simulink model "sampleModel20"  (R2021a)
settings: Solver=VariableStepAuto  StartTime=0.0  StopTime=10.0  RelTol=1e-3
undefined symbols (not defined in the file): DiscIntNeverNeededParam, magnitude, Newton, Raphson
libraries: simulink x274, pid_lib x17
(part 1 of 16)
settings Model: Creator=user  LastModifiedBy=user

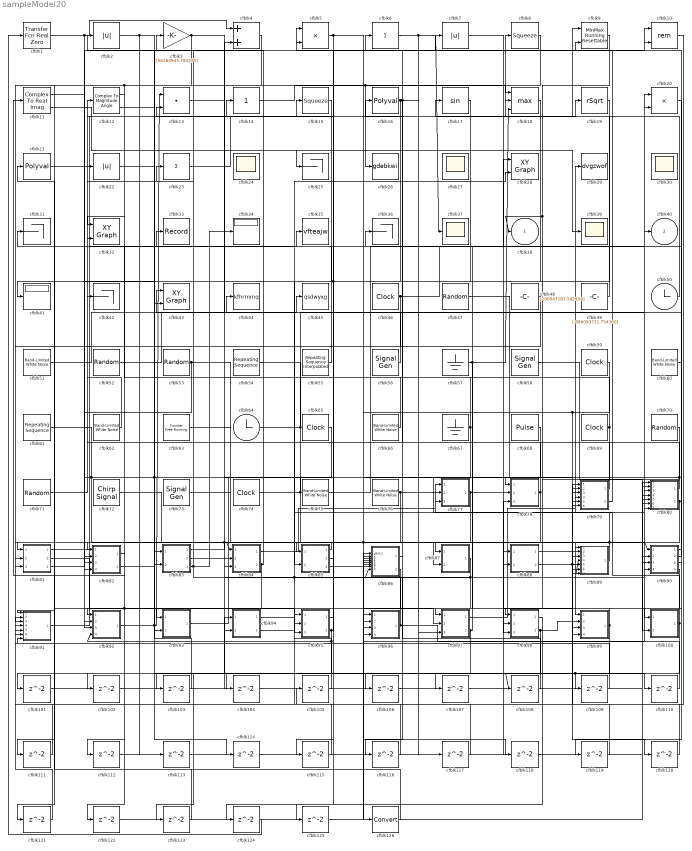
== system sampleModel20 ==
  cfblk1 : simulink/Discrete/Transfer Fcn Real Zero  ZeroZ=0.75  ICPrevInput=0.0  DoSatur=off
      settings: SourceProductBaseCode=SL
  cfblk10 : Math  Operator=rem  SaturateOnIntegerOverflow=on
  cfblk100 : Subsystem
  cfblk{101..125} (25 alike) : Delay  SampleTime=1
  cfblk11 : ComplexToRealImag
  cfblk12 : ComplexToMagnitudeAngle
  cfblk126 : DataTypeConversion
  cfblk13 : DotProduct  InputSameDT=on  OutDataTypeStr=Inherit: Inherit via internal rule
  cfblk14 : simulink/Math Operations/Slider Gain  gain=1  low=0  high=2
  cfblk15 : Squeeze
  cfblk16 : Polyval  Coefs=[ +2.081618890e-019, -1.441693666e-014, +4.719686976e-010, -8.536869453e-006, +1.621573104e-001, -8.087801117e+001 ]
  cfblk17 : Trigonometry
  cfblk18 : MinMax  Function=max  Inputs=3
  cfblk19 : Sqrt  Operator=rSqrt  AlgorithmType=Newton-Raphson  SaturateOnIntegerOverflow=on
  cfblk2 : Abs
  cfblk20 : Product  Inputs=**
  cfblk21 : Polyval  Coefs=[ +2.081618890e-019, -1.441693666e-014, +4.719686976e-010, -8.536869453e-006, +1.621573104e-001, -8.087801117e+001 ]
  cfblk22 : Abs
  cfblk23 : Sum  Inputs=+
  cfblk{24,27,30,37,39} (5 alike) : Scope
      cfblk24 settings: Floating=on
      cfblk27 settings: Floating=on
      cfblk30 settings: Floating=on
  cfblk{25,31,36,42} (4 alike) : Terminator
  cfblk26 : ToWorkspace  VariableName=gdebkwi  SaveFormat=Timeseries  SampleTime=-1
  cfblk28 : simulink/Sinks/XY Graph  xmin=-1  xmax=1  ymin=-1  ymax=1  st=-1
  cfblk29 : ToWorkspace  VariableName=dvgzwof  SaveFormat=Timeseries  SampleTime=-1
  cfblk3 : Gain  Gain=[56264945.784275]
  cfblk32 : simulink/Sinks/XY Graph  xmin=-1  xmax=1  ymin=-1  ymax=1  st=-1
  cfblk33 : Record  FileSettingsInternal="{\"entries\":[{\"content\":{\"excelSettings\":{\"content\":{},\"type\":\"Streamout.ExcelSettings\"}},\"type\":\"Streamout.FileSettingStorage\",\"uuid\":\"928b06ce-2ca3-4e43-b9c9-2fca8fc53509\"}],\"packageUris\":[\"http://schema.mathworks.com/mf0/streamout_blocks/R2020a\"],\"version\":\"1.0\"}"  SignalsInternal="{\"entries\":[{\"content\":{\"signals\":[{\"content\":{\"blockPath\":[\"sampleModel20/cfblk33\"],\"channel\":[],\"dimensions\":[1],\"domain\":\"samplemodel20/cfblk33\",\"lineColor\":\"#77ac30\",\"plots\":[1],\"port\":1,\"sid\":[\"\"],\"signalID\":19970752,\"signalName\":\"cfblk55\"},\"type\":\"RecordBlkView.Signal\",\"uuid\":\"c558b8a0-6107-4ffd-af5c-dee7680296d7\"}]},\"type\":\"RecordBlkView.InputSignals\",\"uuid\":\"2b2755c9-adf7-49b9-84f7-e9e1f548de1f\"}],\"packageUris\":[\"http://schema.mathworks.com/mf0/streamout_blocks/R2020a\"],\"version\":\"1.0\"}"  VisualizationBindings="{\"sparklinesplugin\":{\"info\":[{\"bindingParametersList\":[],\"subplotID\":1}]}}"
  cfblk34 : Display
  cfblk35 : ToWorkspace  VariableName=vfteajw  SaveFormat=Timeseries  SampleTime=-1
  cfblk4 : Sum
  cfblk41 : Display
  cfblk43 : simulink/Sinks/XY Graph  xmin=-1  xmax=1  ymin=-1  ymax=1  st=-1
  cfblk44 : ToWorkspace  VariableName=kfhrmmq  SaveFormat=Timeseries  SampleTime=-1
  cfblk45 : ToWorkspace  VariableName=qsdwyxg  SaveFormat=Timeseries  SampleTime=-1
  cfblk{46,59,65,69,74} (5 alike) : DigitalClock
  cfblk47 : RandomNumber  Mean=[-41753.040388]  Variance=[63915.709445]  Seed=[511170235.000000]  SampleTime=0.1
  cfblk48 : Constant  Value=[200047183.582154]  SampleTime=1
  cfblk49 : Constant  Value=[-886093721.754360]  SampleTime=1
  cfblk5 : Product
  cfblk50 : Clock
  cfblk51 : simulink/Sources/Band-Limited White Noise  Cov=[9193384842.285128]  Ts=0.1  seed=[7756507675.000000]
  cfblk52 : RandomNumber  Mean=[-72813.346888]  Variance=[96356.026322]  Seed=[58960493.000000]  SampleTime=0.1
  cfblk53 : UniformRandomNumber  Minimum=[-6749666358.615873]  Maximum=[6273327936.656572]  Seed=[6207066.000000]  SampleTime=0.1
  cfblk54 : simulink/Sources/Repeating Sequence  rep_seq_t=[0 2]  rep_seq_y=[334719478.211440, -569550998.056046]
  cfblk55 : simulink/Sources/Repeating Sequence Interpolated  OutValues=[101544910.946823, 391282082.256712, 433310399.263298, 204880323.228426, -388511505.652922]  TimeValues=[0 0.1 0.5 0.6 1].'  LookUpMeth=Use Input Nearest  tsamp=0.01  OutMin=[]  OutMax=[]  OutDataTypeStr=double  OutputDataTypeScalingMode=double  OutDataType=fixdt(0,8)  OutScaling=2^-10
  cfblk56 : SignalGenerator  WaveForm=square  Amplitude=[548376924.788326]
  cfblk57 : Ground
  cfblk58 : SignalGenerator  Amplitude=[184204147.684020]
  cfblk6 : Sum  Inputs=+
  cfblk60 : simulink/Sources/Band-Limited White Noise  Cov=[6011912995.701045]  Ts=0.1  seed=[7883111785.000000]
  cfblk61 : simulink/Sources/Repeating Sequence  rep_seq_t=[0 2]  rep_seq_y=[573110201.455736, -888529698.256362]
  cfblk62 : simulink/Sources/Band-Limited White Noise  Cov=[5852828294.400876]  Ts=0.1  seed=[308601692.000000]
  cfblk63 : simulink/Sources/Counter Free-Running  NumBits=[57.000000]  tsamp=-1
  cfblk64 : Clock
  cfblk66 : simulink/Sources/Band-Limited White Noise  Cov=[6955568622.597345]  Ts=0.1  seed=[820560845.000000]
  cfblk67 : Ground
  cfblk68 : DiscretePulseGenerator  PulseType=Time based  Amplitude=[-307176578.790476]  Period=[8696334.995462]  PulseWidth=5  PhaseDelay=[9.000000]
  cfblk7 : Abs
  cfblk70 : UniformRandomNumber  Minimum=[-759248775.546139]  Maximum=[9415666302.746086]  Seed=[58100389.000000]  SampleTime=0.1
  cfblk71 : UniformRandomNumber  Minimum=[-2486475271.173175]  Maximum=[2075060491.074587]  Seed=[20322190.000000]  SampleTime=0.1
  cfblk72 : simulink/Sources/Chirp Signal  f1=[314613710.646437]  T=[-916076924.706605]  f2=[-822624780.040317]
  cfblk73 : SignalGenerator  Amplitude=[415883044.932598]  Units=rad/sec
  cfblk75 : simulink/Sources/Band-Limited White Noise  Cov=[1094535168.541819]  Ts=0.1  seed=[4220656770.000000]
  cfblk76 : simulink/Sources/Band-Limited White Noise  Cov=[7039707520.686424]  Ts=0.1  seed=[3381655650.000000]
  cfblk77 : Subsystem
  cfblk78 : Subsystem
  cfblk79 : Subsystem
  cfblk8 : Squeeze
  cfblk80 : Subsystem
  cfblk81 : Subsystem
  cfblk82 : Subsystem
  cfblk83 : Subsystem
  cfblk84 : Subsystem
  cfblk85 : Subsystem
  cfblk86 : Subsystem
  cfblk87 : Subsystem
  cfblk88 : Subsystem
  cfblk89 : Subsystem
  cfblk9 : simulink/Math Operations/MinMax Running Resettable  Function=min  vinit=0.0
  cfblk90 : Subsystem
  cfblk91 : Subsystem
  cfblk92 : Subsystem
  cfblk93 : Subsystem
  cfblk94 : Subsystem
  cfblk95 : Subsystem
  cfblk96 : Subsystem
  cfblk97 : Subsystem
  cfblk98 : Subsystem
  cfblk99 : Subsystem
  cfblk38 : Outport
  cfblk40 : Outport  Port=2
  wires:
  cfblk74/1 -> cfblk99/1(cfblk1), cfblk79/2(cfblk10)
  cfblk93/1(cfblk2) -> cfblk78/1(cfblk1)
  cfblk96/1(cfblk2) -> cfblk20/1, cfblk3/1
  cfblk90/1(cfblk2) -> cfblk5/1
  cfblk50/1 -> cfblk8/1
  cfblk81/1(cfblk2) -> cfblk35/1
  cfblk8/1 -> cfblk26/1, cfblk81/3(cfblk9)
  cfblk6/1 -> cfblk37/1, cfblk97/3(cfblk6)
  cfblk84/1(cfblk2) -> cfblk77/1(cfblk1)
  cfblk49/1 -> cfblk17/1
  cfblk1/1 -> cfblk4/1, cfblk79/5(cfblk13)
  cfblk71/1 -> cfblk15/1
  cfblk62/1 -> cfblk12/1
  cfblk64/1 -> cfblk20/2, cfblk98/2(cfblk10)
  cfblk3/1 -> cfblk111/1, cfblk112/1, cfblk89/7(cfblk15), cfblk110/1
  cfblk15/1 -> cfblk41/1
  cfblk90/2(cfblk13) -> cfblk36/1
  cfblk84/2(cfblk13) -> cfblk121/1, cfblk122/1, cfblk2/1
  cfblk82/1(cfblk2) -> cfblk11/1
  cfblk92/1(cfblk2) -> cfblk13/1, cfblk107/1
  cfblk87/1(cfblk2) -> cfblk86/8(cfblk16), cfblk102/1
  cfblk67/1 -> cfblk5/2, cfblk86/5(cfblk13)
  cfblk73/1 -> cfblk90/1(cfblk1), cfblk86/4(cfblk12)
  cfblk91/1(cfblk2) -> cfblk19/1
  cfblk56/1 -> cfblk44/1
  cfblk55/1 -> cfblk33/1
  cfblk79/1(cfblk2) -> cfblk16/1
  cfblk89/1(cfblk2) -> cfblk84/1(cfblk1), cfblk79/4(cfblk12)
  cfblk20/1 -> cfblk100/1(cfblk1)
  cfblk4/1 -> cfblk94/2(cfblk12)
  cfblk66/1 -> cfblk23/1
  cfblk85/1(cfblk2) -> cfblk82/1(cfblk1)
  cfblk18/1 -> cfblk96/2(cfblk8)
  cfblk58/1 -> cfblk100/2(cfblk12)
  cfblk52/1 -> cfblk45/1
  cfblk5/1 -> cfblk85/1(cfblk1), cfblk97/2(cfblk5)
  cfblk85/2(cfblk12) -> cfblk13/2
  cfblk23/1 -> cfblk9/1
  cfblk68/1 -> cfblk87/1(cfblk1)
  cfblk99/1(cfblk2) -> cfblk108/1, cfblk109/1, cfblk92/1(cfblk1)
  cfblk97/1(cfblk2) -> cfblk29/1
  cfblk53/1 -> cfblk92/2(cfblk5), cfblk98/3(cfblk11)
  cfblk14/1 -> cfblk18/1
  cfblk46/1 -> cfblk40/1, cfblk91/3(cfblk10)
  cfblk72/1 -> cfblk89/1(cfblk1)
  cfblk78/1(cfblk2) -> cfblk42/1, cfblk81/2(cfblk8)
  cfblk16/1 -> cfblk82/4(cfblk7), cfblk115/1, cfblk116/1, cfblk117/1
  cfblk97/2(cfblk7) -> cfblk31/1, cfblk101/1
  cfblk60/1 -> cfblk10/1
  cfblk21/1 -> cfblk18/2
  cfblk80/1(cfblk2) -> cfblk6/1
  cfblk57/1 -> cfblk18/3, cfblk97/1(cfblk1)
  cfblk70/1 -> cfblk93/1(cfblk1), cfblk88/2(cfblk7)
  cfblk17/1 -> cfblk85/2(cfblk11)
  cfblk59/1 -> cfblk89/5(cfblk13), cfblk89/6(cfblk14), cfblk96/4(cfblk10)
  cfblk12/1 -> cfblk32/1
  cfblk54/1 -> cfblk78/2(cfblk11)
  cfblk9/1 -> cfblk38/1, cfblk98/1(cfblk1)
  cfblk69/1 -> cfblk32/2, cfblk79/3(cfblk11)
  cfblk65/1 -> cfblk84/2(cfblk11)
  cfblk86/1(cfblk2) -> cfblk93/2(cfblk8)
  cfblk81/2(cfblk10) -> cfblk95/3(cfblk13)
  cfblk79/2(cfblk15) -> cfblk7/1
  cfblk51/1 -> cfblk4/2
  cfblk88/1(cfblk2) -> cfblk90/3(cfblk11)
  cfblk22/1 -> cfblk84/3(cfblk12)
  cfblk81/3(cfblk11) -> cfblk9/2
  cfblk75/1 -> cfblk28/1
  cfblk12/2 -> cfblk25/1
  cfblk2/1 -> cfblk79/6(cfblk14), cfblk114/1, cfblk113/1
  cfblk98/2(cfblk12) -> cfblk99/2(cfblk8), cfblk125/1
  cfblk80/2(cfblk13) -> cfblk43/1, cfblk91/1(cfblk1)
  cfblk19/1 -> cfblk83/2(cfblk8)
  cfblk83/1(cfblk2) -> cfblk87/2(cfblk10)
  cfblk76/1 -> cfblk81/1(cfblk1), cfblk80/7(cfblk12)
  cfblk61/1 -> cfblk89/2(cfblk10), cfblk77/2(cfblk11)
  cfblk90/4(cfblk15) -> cfblk99/3(cfblk9)
  cfblk95/2(cfblk14) -> cfblk92/4(cfblk7), cfblk123/1, cfblk14/1
  cfblk82/2(cfblk8) -> cfblk10/2
  cfblk100/1(cfblk2) -> cfblk77/3(cfblk12), cfblk104/1
  cfblk77/1(cfblk2) -> cfblk82/2(cfblk5), cfblk99/4(cfblk10)
  cfblk48/1 -> cfblk82/3(cfblk6)
  cfblk47/1 -> cfblk89/3(cfblk11)
  cfblk7/1 -> cfblk88/1(cfblk1)
  cfblk83/2(cfblk9) -> cfblk90/4(cfblk12)
  cfblk94/1(cfblk2) -> cfblk80/3(cfblk8)
  cfblk94/2(cfblk13) -> cfblk28/2, cfblk89/4(cfblk12)
  cfblk86/2(cfblk17) -> cfblk92/3(cfblk6)
  cfblk83/3(cfblk10) -> cfblk22/1, cfblk34/1
  cfblk11/1 -> cfblk43/2
  cfblk11/2 -> cfblk39/1
  cfblk101/1 -> cfblk80/4(cfblk9)
  cfblk102/1 -> cfblk94/1(cfblk1)
  cfblk95/1(cfblk2) -> cfblk103/1
  cfblk103/1 -> cfblk83/1(cfblk1)
  cfblk104/1 -> cfblk86/1(cfblk1)
  cfblk10/1 -> cfblk105/1
  cfblk105/1 -> cfblk95/1(cfblk1)
  cfblk13/1 -> cfblk106/1
  cfblk106/1 -> cfblk80/1(cfblk1)
  cfblk107/1 -> cfblk80/5(cfblk10)
  cfblk108/1 -> cfblk86/3(cfblk11)
  cfblk109/1 -> cfblk91/6(cfblk13)
  cfblk110/1 -> cfblk96/1(cfblk1)
  cfblk111/1 -> cfblk91/2(cfblk9)
  cfblk112/1 -> cfblk86/6(cfblk14)
  cfblk113/1 -> cfblk80/2(cfblk7)
  cfblk114/1 -> cfblk78/3(cfblk12)
  cfblk115/1 -> cfblk95/2(cfblk12)
  cfblk116/1 -> cfblk86/2(cfblk10)
  cfblk117/1 -> cfblk91/5(cfblk12)
  cfblk85/3(cfblk13) -> cfblk118/1
  cfblk118/1 -> cfblk90/2(cfblk10)
  cfblk90/3(cfblk14) -> cfblk119/1
  cfblk119/1 -> cfblk96/3(cfblk9)
  cfblk88/2(cfblk8) -> cfblk120/1
  cfblk120/1 -> cfblk79/1(cfblk1)
  cfblk121/1 -> cfblk91/4(cfblk11)
  cfblk122/1 -> cfblk80/6(cfblk11)
  cfblk123/1 -> cfblk91/7(cfblk14)
  cfblk98/1(cfblk2) -> cfblk124/1
  cfblk124/1 -> cfblk1/1
  cfblk125/1 -> cfblk86/7(cfblk15)
  cfblk63/1 -> cfblk126/1
  cfblk126/1 -> cfblk21/1

== system sampleModel20/cfblk100 ==
  cfblk1 : Inport
  cfblk12 : Inport  Port=2
  cfblk10 : Subsystem
  cfblk11 : Subsystem
  cfblk{13..19} (7 alike) : Delay  SampleTime=1
  cfblk3 : DiscreteFir  SampleTime=1
  cfblk4 : Product
  cfblk5 : Bias  Bias=[44627423.710003]
  cfblk6 : Sin  TimeSource=Use external signal  SampleTime=0
  cfblk7 : Subsystem
  cfblk8 : Subsystem
  cfblk9 : Subsystem
  cfblk2 : Outport
  wires:
  cfblk7/1(cfblk2) -> cfblk5/1
  cfblk1/1 -> cfblk7/1(cfblk1), cfblk8/2(cfblk11)
  cfblk12/1 -> cfblk10/1(cfblk1)
  cfblk5/1 -> cfblk6/1, cfblk11/2(cfblk9)
  cfblk9/1(cfblk2) -> cfblk3/1
  cfblk3/1 -> cfblk8/3(cfblk12), cfblk18/1
  cfblk9/2(cfblk12) -> cfblk4/1, cfblk19/1
  cfblk8/1(cfblk2) -> cfblk2/1, cfblk17/1
  cfblk6/1 -> cfblk11/1(cfblk1), cfblk10/2(cfblk4), cfblk15/1, cfblk16/1
  cfblk4/1 -> cfblk8/1(cfblk1)
  cfblk11/1(cfblk2) -> cfblk13/1, cfblk14/1
  cfblk10/1(cfblk2) -> cfblk4/2
  cfblk10/2(cfblk6) -> cfblk9/2(cfblk10)
  cfblk10/3(cfblk7) -> cfblk9/3(cfblk11)
  cfblk13/1 -> cfblk7/3(cfblk5)
  cfblk14/1 -> cfblk7/6(cfblk8)
  cfblk15/1 -> cfblk7/4(cfblk6)
  cfblk16/1 -> cfblk7/5(cfblk7)
  cfblk17/1 -> cfblk7/2(cfblk4)
  cfblk18/1 -> cfblk9/1(cfblk1)
  cfblk19/1 -> cfblk10/3(cfblk5)

== system sampleModel20/cfblk77 ==
  cfblk1 : Inport
  cfblk11 : Inport  Port=2
  cfblk12 : Inport  Port=3
  cfblk10 : Subsystem
  cfblk{13..23} (11 alike) : Delay  SampleTime=1
  cfblk3 : Polyval  Coefs=[ +2.081618890e-019, -1.441693666e-014, +4.719686976e-010, -8.536869453e-006, +1.621573104e-001, -8.087801117e+001 ]
  cfblk4 : Subsystem
  cfblk5 : Subsystem
  cfblk6 : Subsystem
  cfblk7 : Subsystem
  cfblk8 : Subsystem
  cfblk9 : Subsystem
  cfblk2 : Outport
  wires:
  cfblk9/1(cfblk2) -> cfblk5/4(cfblk13), cfblk13/1
  cfblk10/1(cfblk2) -> cfblk4/3(cfblk8), cfblk20/1, cfblk21/1
  cfblk4/1(cfblk2) -> cfblk17/1, cfblk18/1, cfblk19/1
  cfblk8/1(cfblk2) -> cfblk7/1(cfblk1)
  cfblk11/1 -> cfblk7/2(cfblk11), cfblk5/5(cfblk14)
  cfblk6/1(cfblk2) -> cfblk2/1, cfblk9/4(cfblk10), cfblk5/3(cfblk12)
  cfblk7/1(cfblk2) -> cfblk4/2(cfblk7), cfblk16/1
  cfblk3/1 -> cfblk10/1(cfblk1)
  cfblk12/1 -> cfblk8/2(cfblk11), cfblk8/4(cfblk13), cfblk5/1(cfblk1)
  cfblk5/3(cfblk17) -> cfblk8/3(cfblk12), cfblk23/1
  cfblk8/2(cfblk14) -> cfblk4/1(cfblk1)
  cfblk1/1 -> cfblk6/3(cfblk11)
  cfblk8/3(cfblk15) -> cfblk10/2(cfblk8), cfblk3/1, cfblk22/1
  cfblk13/1 -> cfblk6/1(cfblk1)
  cfblk5/1(cfblk2) -> cfblk14/1
  cfblk14/1 -> cfblk9/1(cfblk1)
  cfblk5/2(cfblk16) -> cfblk15/1
  cfblk15/1 -> cfblk9/3(cfblk9)
  cfblk16/1 -> cfblk8/1(cfblk1)
  cfblk17/1 -> cfblk6/2(cfblk10)
  cfblk18/1 -> cfblk6/4(cfblk12)
  cfblk19/1 -> cfblk5/2(cfblk11)
  cfblk20/1 -> cfblk9/2(cfblk8)
  cfblk21/1 -> cfblk9/5(cfblk11)
  cfblk22/1 -> cfblk5/6(cfblk15)
  cfblk23/1 -> cfblk6/5(cfblk13)

== system sampleModel20/cfblk78 ==
  cfblk1 : Inport
  cfblk11 : Inport  Port=2
  cfblk12 : Inport  Port=3
  cfblk10 : Subsystem
  cfblk{13..17} (5 alike) : Delay  SampleTime=1
  cfblk3 : simulink/Math Operations/MinMax Running Resettable  Function=min  vinit=0.0
  cfblk4 : Gain  Gain=[460184009.400901]
  cfblk5 : Sum  Inputs=+-
  cfblk6 : Product  Inputs=*
  cfblk7 : Subsystem
  cfblk8 : Subsystem
  cfblk9 : Subsystem
  cfblk2 : Outport
  wires:
  cfblk5/1 -> cfblk10/1(cfblk1)
  cfblk12/1 -> cfblk6/1, cfblk8/3(cfblk8), cfblk5/2
  cfblk9/1(cfblk2) -> cfblk7/1(cfblk1)
  cfblk11/1 -> cfblk2/1, cfblk5/1
  cfblk10/1(cfblk2) -> cfblk3/1
  cfblk1/1 -> cfblk7/2(cfblk8), cfblk10/3(cfblk10)
  cfblk8/1(cfblk2) -> cfblk3/2, cfblk14/1
  cfblk6/1 -> cfblk10/2(cfblk9), cfblk10/5(cfblk12), cfblk8/5(cfblk10)
  cfblk7/1(cfblk2) -> cfblk4/1, cfblk8/2(cfblk7)
  cfblk9/2(cfblk13) -> cfblk8/1(cfblk1), cfblk8/4(cfblk9), cfblk17/1
  cfblk10/2(cfblk13) -> cfblk9/1(cfblk1)
  cfblk3/1 -> cfblk15/1, cfblk16/1
  cfblk4/1 -> cfblk13/1
  cfblk13/1 -> cfblk7/4(cfblk10)
  cfblk14/1 -> cfblk7/3(cfblk9)
  cfblk15/1 -> cfblk7/5(cfblk11)
  cfblk16/1 -> cfblk7/6(cfblk12)
  cfblk17/1 -> cfblk10/4(cfblk11)

== system sampleModel20/cfblk79 ==
  cfblk1 : Inport
  cfblk10 : Inport  Port=2
  cfblk11 : Inport  Port=3
  cfblk12 : Inport  Port=4
  cfblk13 : Inport  Port=5
  cfblk14 : Inport  Port=6
  cfblk16 : Delay  SampleTime=1
  cfblk17 : Delay  SampleTime=1
  cfblk3 : UnaryMinus
  cfblk4 : Rounding
  cfblk5 : Reshape
  cfblk6 : Bias  Bias=[-187698543.818652]
  cfblk7 : Sum  Inputs=--
  cfblk8 : Subsystem
  cfblk9 : Subsystem
  cfblk2 : Outport
  cfblk15 : Outport  Port=2
  wires:
  cfblk1/1 -> cfblk5/1
  cfblk12/1 -> cfblk2/1
  cfblk10/1 -> cfblk6/1
  cfblk11/1 -> cfblk15/1
  cfblk7/1 -> cfblk3/1, cfblk9/4(cfblk11)
  cfblk5/1 -> cfblk8/1(cfblk1)
  cfblk14/1 -> cfblk4/1
  cfblk13/1 -> cfblk7/1
  cfblk4/1 -> cfblk9/1(cfblk1)
  cfblk6/1 -> cfblk9/2(cfblk9)
  cfblk8/1(cfblk2) -> cfblk9/3(cfblk10)
  cfblk8/2(cfblk8) -> cfblk7/2
  cfblk9/1(cfblk2) -> cfblk16/1
  cfblk16/1 -> cfblk8/2(cfblk6)
  cfblk3/1 -> cfblk17/1
  cfblk17/1 -> cfblk8/3(cfblk7)

== system sampleModel20/cfblk80 ==
  cfblk1 : Inport
  cfblk7 : Inport  Port=2
  cfblk8 : Inport  Port=3
  cfblk9 : Inport  Port=4
  cfblk10 : Inport  Port=5
  cfblk11 : Inport  Port=6
  cfblk12 : Inport  Port=7
  cfblk3 : DotProduct  InputSameDT=on  OutDataTypeStr=Inherit: Inherit via internal rule
  cfblk4 : Signum
  cfblk5 : Sin  TimeSource=Use external signal  SampleTime=0
  cfblk6 : Subsystem
  cfblk2 : Outport
  cfblk13 : Outport  Port=2
  wires:
  cfblk7/1 -> cfblk13/1
  cfblk3/1 -> cfblk6/1(cfblk1)
  cfblk5/1 -> cfblk4/1
  cfblk8/1 -> cfblk3/1
  cfblk4/1 -> cfblk6/2(cfblk9)
  cfblk11/1 -> cfblk5/1
  cfblk9/1 -> cfblk3/2
  cfblk10/1 -> cfblk6/3(cfblk10), cfblk6/5(cfblk12)
  cfblk1/1 -> cfblk6/4(cfblk11)
  cfblk12/1 -> cfblk2/1

== system sampleModel20/cfblk81 ==
  cfblk1 : Inport
  cfblk8 : Inport  Port=2
  cfblk9 : Inport  Port=3
  cfblk{12..18} (7 alike) : Delay  SampleTime=1
  cfblk3 : Polyval  Coefs=[ +2.081618890e-019, -1.441693666e-014, +4.719686976e-010, -8.536869453e-006, +1.621573104e-001, -8.087801117e+001 ]
  cfblk4 : Subsystem
  cfblk5 : Subsystem
  cfblk6 : Subsystem
  cfblk7 : Subsystem
  cfblk2 : Outport
  cfblk10 : Outport  Port=2
  cfblk11 : Outport  Port=3
  wires:
  cfblk8/1 -> cfblk10/1, cfblk6/1(cfblk1)
  cfblk5/1(cfblk2) -> cfblk4/1(cfblk1)
  cfblk9/1 -> cfblk7/1(cfblk1), cfblk7/4(cfblk12), cfblk4/4(cfblk15), cfblk6/4(cfblk10)
  cfblk5/2(cfblk8) -> cfblk11/1, cfblk18/1
  cfblk3/1 -> cfblk2/1, cfblk13/1, cfblk14/1, cfblk15/1
  cfblk4/1(cfblk2) -> cfblk6/3(cfblk9), cfblk12/1
  cfblk6/1(cfblk2) -> cfblk3/1, cfblk16/1, cfblk17/1
  cfblk1/1 -> cfblk7/3(cfblk11)
  cfblk7/1(cfblk2) -> cfblk5/1(cfblk1)
  cfblk7/2(cfblk14) -> cfblk5/2(cfblk5)
  cfblk7/3(cfblk15) -> cfblk4/2(cfblk13), cfblk6/5(cfblk11)
  cfblk12/1 -> cfblk7/2(cfblk10)
  cfblk13/1 -> cfblk4/3(cfblk14)
  cfblk14/1 -> cfblk5/3(cfblk6)
  cfblk15/1 -> cfblk6/2(cfblk8)
  cfblk16/1 -> cfblk4/5(cfblk16)
  cfblk17/1 -> cfblk5/4(cfblk7)
  cfblk18/1 -> cfblk7/5(cfblk13)

== system sampleModel20/cfblk82 ==
  cfblk1 : Inport
  cfblk5 : Inport  Port=2
  cfblk6 : Inport  Port=3
  cfblk7 : Inport  Port=4
  cfblk3 : Trigonometry
  cfblk4 : Subsystem
  cfblk2 : Outport
  cfblk8 : Outport  Port=2
  wires:
  cfblk1/1 -> cfblk4/1(cfblk1), cfblk4/3(cfblk14)
  cfblk5/1 -> cfblk8/1
  cfblk7/1 -> cfblk3/1
  cfblk6/1 -> cfblk4/2(cfblk13)
  cfblk3/1 -> cfblk2/1, cfblk4/4(cfblk15)

== system sampleModel20/cfblk83 ==
  cfblk1 : Inport
  cfblk8 : Inport  Port=2
  cfblk{11..15} (5 alike) : Delay  SampleTime=1
  cfblk3 : UnaryMinus
  cfblk4 : Subsystem
  cfblk5 : Subsystem
  cfblk6 : Subsystem
  cfblk7 : Subsystem
  cfblk2 : Outport
  cfblk9 : Outport  Port=2
  cfblk10 : Outport  Port=3
  wires:
  cfblk3/1 -> cfblk10/1, cfblk4/1(cfblk1), cfblk4/3(cfblk10), cfblk4/5(cfblk12)
  cfblk5/1(cfblk2) -> cfblk2/1
  cfblk8/1 -> cfblk5/1(cfblk1), cfblk7/5(cfblk15), cfblk7/6(cfblk16)
  cfblk4/2(cfblk13) -> cfblk9/1
  cfblk1/1 -> cfblk7/1(cfblk1)
  cfblk7/1(cfblk2) -> cfblk5/3(cfblk8), cfblk4/2(cfblk9), cfblk4/4(cfblk11)
  cfblk6/2(cfblk7) -> cfblk3/1, cfblk13/1, cfblk14/1
  cfblk5/2(cfblk9) -> cfblk6/1(cfblk1)
  cfblk5/3(cfblk10) -> cfblk6/2(cfblk6)
  cfblk6/1(cfblk2) -> cfblk11/1
  cfblk11/1 -> cfblk7/2(cfblk12)
  cfblk4/1(cfblk2) -> cfblk12/1
  cfblk12/1 -> cfblk5/2(cfblk7)
  cfblk13/1 -> cfblk7/4(cfblk14)
  cfblk14/1 -> cfblk7/7(cfblk17)
  cfblk5/4(cfblk11) -> cfblk15/1
  cfblk15/1 -> cfblk7/3(cfblk13)

== system sampleModel20/cfblk84 ==
  cfblk1 : Inport
  cfblk11 : Inport  Port=2
  cfblk12 : Inport  Port=3
  cfblk10 : Subsystem
  cfblk{14..25} (12 alike) : Delay  SampleTime=1
  cfblk3 : MinMax  Function=max  Inputs=2
  cfblk4 : Abs
  cfblk5 : Subsystem
  cfblk6 : Subsystem
  cfblk7 : Subsystem
  cfblk8 : Subsystem
  cfblk9 : Subsystem
  cfblk2 : Outport
  cfblk13 : Outport  Port=2
  wires:
  cfblk1/1 -> cfblk7/1(cfblk1)
  cfblk9/1(cfblk2) -> cfblk2/1
  cfblk12/1 -> cfblk8/1(cfblk1), cfblk8/2(cfblk10)
  cfblk4/1 -> cfblk10/2(cfblk12), cfblk5/4(cfblk12), cfblk7/6(cfblk15)
  cfblk9/3(cfblk11) -> cfblk19/1, cfblk20/1
  cfblk11/1 -> cfblk4/1, cfblk9/2(cfblk8), cfblk7/5(cfblk14), cfblk8/5(cfblk13)
  cfblk8/1(cfblk2) -> cfblk5/1(cfblk1), cfblk5/3(cfblk11), cfblk9/3(cfblk9), cfblk22/1
  cfblk5/2(cfblk13) -> cfblk16/1, cfblk17/1
  cfblk3/1 -> cfblk5/2(cfblk10)
  cfblk10/1(cfblk2) -> cfblk6/3(cfblk8), cfblk24/1, cfblk25/1
  cfblk7/1(cfblk2) -> cfblk10/5(cfblk15)
  cfblk6/2(cfblk9) -> cfblk3/1
  cfblk6/3(cfblk10) -> cfblk9/1(cfblk1), cfblk8/4(cfblk12), cfblk21/1, cfblk23/1
  cfblk7/2(cfblk17) -> cfblk13/1, cfblk8/3(cfblk11)
  cfblk6/1(cfblk2) -> cfblk14/1
  cfblk14/1 -> cfblk10/1(cfblk1)
  cfblk5/1(cfblk2) -> cfblk15/1
  cfblk15/1 -> cfblk6/2(cfblk7)
  cfblk16/1 -> cfblk10/4(cfblk14)
  cfblk17/1 -> cfblk3/2
  cfblk9/2(cfblk10) -> cfblk18/1
  cfblk18/1 -> cfblk6/1(cfblk1)
  cfblk19/1 -> cfblk10/3(cfblk13)
  cfblk20/1 -> cfblk7/2(cfblk11)
  cfblk21/1 -> cfblk10/7(cfblk17)
  cfblk22/1 -> cfblk10/6(cfblk16)
  cfblk23/1 -> cfblk7/7(cfblk16)
  cfblk24/1 -> cfblk7/3(cfblk12)
  cfblk25/1 -> cfblk7/4(cfblk13)

== system sampleModel20/cfblk85 ==
  cfblk1 : Inport
  cfblk11 : Inport  Port=2
  cfblk10 : Subsystem
  cfblk14 : Delay  SampleTime=1
  cfblk15 : Delay  SampleTime=1
  cfblk3 : Product  Inputs=*
  cfblk4 : Sum  Inputs=+-
  cfblk5 : ComplexToRealImag
  cfblk6 : Polyval  Coefs=[ +2.081618890e-019, -1.441693666e-014, +4.719686976e-010, -8.536869453e-006, +1.621573104e-001, -8.087801117e+001 ]
  cfblk7 : Rounding
  cfblk8 : Sum  Inputs=|++
  cfblk9 : Subsystem
  cfblk2 : Outport
  cfblk12 : Outport  Port=2
  cfblk13 : Outport  Port=3
  wires:
  cfblk1/1 -> cfblk3/1, cfblk10/3(cfblk8)
  cfblk6/1 -> cfblk7/1, cfblk8/1, cfblk10/2(cfblk7)
  cfblk9/1(cfblk2) -> cfblk13/1
  cfblk11/1 -> cfblk2/1, cfblk9/4(cfblk12)
  cfblk5/1 -> cfblk4/1
  cfblk3/1 -> cfblk6/1, cfblk9/3(cfblk11)
  cfblk8/1 -> cfblk9/1(cfblk1), cfblk15/1
  cfblk5/2 -> cfblk4/2, cfblk9/2(cfblk10)
  cfblk7/1 -> cfblk12/1, cfblk10/5(cfblk10), cfblk10/6(cfblk11)
  cfblk10/1(cfblk2) -> cfblk5/1, cfblk8/2
  cfblk4/1 -> cfblk14/1
  cfblk14/1 -> cfblk10/1(cfblk1)
  cfblk15/1 -> cfblk10/4(cfblk9)

== system sampleModel20/cfblk86 ==
  cfblk1 : Inport
  cfblk10 : Inport  Port=2
  cfblk11 : Inport  Port=3
  cfblk12 : Inport  Port=4
  cfblk13 : Inport  Port=5
  cfblk14 : Inport  Port=6
  cfblk15 : Inport  Port=7
  cfblk16 : Inport  Port=8
  cfblk3 : Bias  Bias=[167054584.816413]
  cfblk4 : Polyval  Coefs=[ +2.081618890e-019, -1.441693666e-014, +4.719686976e-010, -8.536869453e-006, +1.621573104e-001, -8.087801117e+001 ]
  cfblk5 : ComplexToRealImag
  cfblk6 : Sum  Inputs=--
  cfblk7 : Trigonometry
  cfblk8 : Subsystem
  cfblk9 : Subsystem
  cfblk2 : Outport
  cfblk17 : Outport  Port=2
  wires:
  cfblk8/1(cfblk2) -> cfblk17/1
  cfblk12/1 -> cfblk2/1, cfblk9/6(cfblk15)
  cfblk13/1 -> cfblk9/1(cfblk1)
  cfblk16/1 -> cfblk6/1
  cfblk1/1 -> cfblk4/1
  cfblk15/1 -> cfblk9/2(cfblk11)
  cfblk3/1 -> cfblk9/3(cfblk12)
  cfblk7/1 -> cfblk8/1(cfblk1)
  cfblk14/1 -> cfblk7/1, cfblk3/1
  cfblk4/1 -> cfblk9/4(cfblk13)
  cfblk11/1 -> cfblk5/1
  cfblk10/1 -> cfblk8/2(cfblk4)
  cfblk6/1 -> cfblk8/3(cfblk5)
  cfblk5/1 -> cfblk9/5(cfblk14)
  cfblk9/1(cfblk2) -> cfblk8/4(cfblk6)
  cfblk9/2(cfblk16) -> cfblk8/5(cfblk7)
  cfblk5/2 -> cfblk6/2

== system sampleModel20/cfblk87 ==
  cfblk1 : Inport
  cfblk10 : Inport  Port=2
  cfblk{11..25} (15 alike) : Delay  SampleTime=1
  cfblk3 : DiscreteZeroPole  Poles=[0 0.5]  Gain=1
  cfblk4 : Sum  Inputs=|++
  cfblk5 : Subsystem
  cfblk6 : Subsystem
  cfblk7 : Subsystem
  cfblk8 : Subsystem
  cfblk9 : Subsystem
  cfblk2 : Outport
  wires:
  cfblk1/1 -> cfblk8/1(cfblk1), cfblk4/2
  cfblk8/1(cfblk2) -> cfblk5/1(cfblk1)
  cfblk8/2(cfblk12) -> cfblk7/1(cfblk1)
  cfblk7/1(cfblk2) -> cfblk9/2(cfblk9)
  cfblk4/1 -> cfblk6/3(cfblk14), cfblk17/1, cfblk18/1, cfblk22/1, cfblk23/1
  cfblk3/1 -> cfblk11/1, cfblk12/1, cfblk13/1, cfblk14/1, cfblk15/1, cfblk16/1
  cfblk5/1(cfblk2) -> cfblk7/4(cfblk15)
  cfblk6/2(cfblk15) -> cfblk20/1, cfblk21/1
  cfblk9/1(cfblk2) -> cfblk3/1
  cfblk10/1 -> cfblk6/1(cfblk1)
  cfblk9/2(cfblk14) -> cfblk4/1
  cfblk9/3(cfblk15) -> cfblk24/1, cfblk25/1
  cfblk8/3(cfblk13) -> cfblk2/1, cfblk6/2(cfblk13)
  cfblk11/1 -> cfblk7/3(cfblk14)
  cfblk12/1 -> cfblk8/3(cfblk9)
  cfblk13/1 -> cfblk8/4(cfblk10)
  cfblk14/1 -> cfblk5/5(cfblk15)
  cfblk15/1 -> cfblk9/6(cfblk13)
  cfblk16/1 -> cfblk8/5(cfblk11)
  cfblk17/1 -> cfblk7/2(cfblk13)
  cfblk18/1 -> cfblk9/4(cfblk11)
  cfblk6/1(cfblk2) -> cfblk19/1
  cfblk19/1 -> cfblk9/1(cfblk1)
  cfblk20/1 -> cfblk9/3(cfblk10)
  cfblk21/1 -> cfblk5/2(cfblk12)
  cfblk22/1 -> cfblk9/5(cfblk12)
  cfblk23/1 -> cfblk5/4(cfblk14)
  cfblk24/1 -> cfblk8/2(cfblk8)
  cfblk25/1 -> cfblk5/3(cfblk13)

== system sampleModel20/cfblk88 ==
  cfblk1 : Inport
  cfblk7 : Inport  Port=2
  cfblk10 : Delay  SampleTime=1
  cfblk11 : Delay  SampleTime=1
  cfblk3 : Sqrt  SaturateOnIntegerOverflow=on
  cfblk4 : Math  Operator=log10  SaturateOnIntegerOverflow=on
  cfblk5 : Subsystem
  cfblk6 : Subsystem
  cfblk9 : Delay  SampleTime=1
  cfblk2 : Outport
  cfblk8 : Outport  Port=2
  wires:
  cfblk6/1(cfblk2) -> cfblk4/1
  cfblk7/1 -> cfblk3/1, cfblk8/1, cfblk6/7(cfblk15)
  cfblk3/1 -> cfblk6/2(cfblk10), cfblk5/2(cfblk9)
  cfblk1/1 -> cfblk6/3(cfblk11), cfblk6/5(cfblk13), cfblk6/8(cfblk16)
  cfblk4/1 -> cfblk2/1, cfblk9/1, cfblk10/1
  cfblk6/2(cfblk17) -> cfblk5/1(cfblk1)
  cfblk9/1 -> cfblk6/4(cfblk12)
  cfblk10/1 -> cfblk6/6(cfblk14)
  cfblk5/1(cfblk2) -> cfblk11/1
  cfblk11/1 -> cfblk6/1(cfblk1)

== system sampleModel20/cfblk89 ==
  cfblk1 : Inport
  cfblk10 : Inport  Port=2
  cfblk11 : Inport  Port=3
  cfblk12 : Inport  Port=4
  cfblk13 : Inport  Port=5
  cfblk14 : Inport  Port=6
  cfblk15 : Inport  Port=7
  cfblk16 : Delay  SampleTime=1
  cfblk17 : Delay  SampleTime=1
  cfblk3 : PermuteDimensions
  cfblk4 : simulink/Math Operations/MinMax Running Resettable  Function=min  vinit=0.0
  cfblk5 : Reshape
  cfblk6 : ComplexToMagnitudeAngle
  cfblk7 : Subsystem
  cfblk8 : Subsystem
  cfblk9 : Subsystem
  cfblk2 : Outport
  wires:
  cfblk7/1(cfblk2) -> cfblk2/1
  cfblk1/1 -> cfblk8/1(cfblk1)
  cfblk5/1 -> cfblk3/1
  cfblk13/1 -> cfblk7/1(cfblk1)
  cfblk12/1 -> cfblk5/1
  cfblk11/1 -> cfblk8/2(cfblk10)
  cfblk9/1(cfblk2) -> cfblk4/1
  cfblk4/1 -> cfblk6/1
  cfblk3/1 -> cfblk4/2
  cfblk7/2(cfblk9) -> cfblk9/2(cfblk9)
  cfblk8/1(cfblk2) -> cfblk9/3(cfblk10)
  cfblk10/1 -> cfblk7/2(cfblk7)
  cfblk14/1 -> cfblk7/3(cfblk8)
  cfblk15/1 -> cfblk9/5(cfblk12)
  cfblk6/1 -> cfblk16/1
  cfblk16/1 -> cfblk9/1(cfblk1)
  cfblk6/2 -> cfblk17/1
  cfblk17/1 -> cfblk9/4(cfblk11)

== system sampleModel20/cfblk90 ==
  cfblk1 : Inport
  cfblk10 : Inport  Port=2
  cfblk11 : Inport  Port=3
  cfblk12 : Inport  Port=4
  cfblk16 : Delay  SampleTime=1
  cfblk17 : Delay  SampleTime=1
  cfblk18 : Delay  SampleTime=1
  cfblk3 : Sum  Inputs=|++
  cfblk4 : Abs
  cfblk5 : Product  Inputs=*
  cfblk6 : UnaryMinus
  cfblk7 : Sin  TimeSource=Use external signal  SampleTime=0
  cfblk8 : Subsystem
  cfblk9 : Subsystem
  cfblk2 : Outport
  cfblk13 : Outport  Port=2
  cfblk14 : Outport  Port=3
  cfblk15 : Outport  Port=4
  wires:
  cfblk12/1 -> cfblk15/1
  cfblk1/1 -> cfblk6/1
  cfblk7/1 -> cfblk14/1
  cfblk8/1(cfblk2) -> cfblk13/1
  cfblk9/1(cfblk2) -> cfblk4/1
  cfblk9/2(cfblk16) -> cfblk5/1
  cfblk10/1 -> cfblk3/1, cfblk9/3(cfblk12), cfblk9/4(cfblk13), cfblk8/4(cfblk8), cfblk8/6(cfblk10)
  cfblk3/1 -> cfblk2/1, cfblk16/1
  cfblk8/2(cfblk11) -> cfblk3/2, cfblk17/1
  cfblk5/1 -> cfblk7/1, cfblk18/1
  cfblk6/1 -> cfblk9/1(cfblk1)
  cfblk9/3(cfblk17) -> cfblk8/1(cfblk1), cfblk8/5(cfblk9)
  cfblk11/1 -> cfblk9/2(cfblk11)
  cfblk4/1 -> cfblk8/2(cfblk6)
  cfblk16/1 -> cfblk8/3(cfblk7)
  cfblk17/1 -> cfblk9/6(cfblk15)
  cfblk18/1 -> cfblk9/5(cfblk14)

== system sampleModel20/cfblk91 ==
  cfblk1 : Inport
  cfblk9 : Inport  Port=2
  cfblk10 : Inport  Port=3
  cfblk11 : Inport  Port=4
  cfblk12 : Inport  Port=5
  cfblk13 : Inport  Port=6
  cfblk14 : Inport  Port=7
  cfblk15 : Delay  SampleTime=1
  cfblk16 : Delay  SampleTime=1
  cfblk17 : Delay  SampleTime=1
  cfblk3 : Rounding
  cfblk4 : DotProduct  InputSameDT=on  OutDataTypeStr=Inherit: Inherit via internal rule
  cfblk5 : Subsystem
  cfblk6 : Subsystem
  cfblk7 : Subsystem
  cfblk8 : Subsystem
  cfblk2 : Outport
  wires:
  cfblk3/1 -> cfblk5/1(cfblk1)
  cfblk7/1(cfblk2) -> cfblk5/2(cfblk11)
  cfblk14/1 -> cfblk2/1
  cfblk12/1 -> cfblk3/1, cfblk8/5(cfblk12)
  cfblk10/1 -> cfblk4/1
  cfblk11/1 -> cfblk6/1(cfblk1)
  cfblk6/2(cfblk10) -> cfblk8/1(cfblk1)
  cfblk7/2(cfblk8) -> cfblk6/2(cfblk7)
  cfblk13/1 -> cfblk4/2
  cfblk9/1 -> cfblk8/2(cfblk9)
  cfblk4/1 -> cfblk6/4(cfblk9)
  cfblk1/1 -> cfblk7/3(cfblk7)
  cfblk6/3(cfblk11) -> cfblk8/3(cfblk10), cfblk8/4(cfblk11)
  cfblk5/1(cfblk2) -> cfblk15/1
  cfblk15/1 -> cfblk7/2(cfblk6)
  cfblk6/1(cfblk2) -> cfblk16/1
  cfblk16/1 -> cfblk7/1(cfblk1)
  cfblk8/1(cfblk2) -> cfblk17/1
  cfblk17/1 -> cfblk6/3(cfblk8)

== system sampleModel20/cfblk92 ==
  cfblk1 : Inport
  cfblk5 : Inport  Port=2
  cfblk6 : Inport  Port=3
  cfblk7 : Inport  Port=4
  cfblk3 : pid_lib/PID Controller  Controller=PID  Form=Parallel  TimeDomain=Discrete-time  UseExternalTs=off  SampleTime=1  IntegratorMethod=Forward Euler  FilterMethod=Forward Euler  ControllerParametersSource=internal  P=1  I=1  D=0  UseFilter=on  N=100  TunerSelectOption=Transfer Function Based (PID Tuner App)  InitialConditionSource=internal  InitialConditionForIntegrator=0  InitialConditionForFilter=0  DifferentiatorICPrevScaledInput=0  ExternalReset=none  TrackingMode=off  Kt=1  LimitOutput=off  SatLimitsSource=internal  UpperSaturationLimit=inf  LowerSaturationLimit=-inf  LinearizeAsGain=off  AntiWindupMode=none  Kb=1  POutMin=[]  POutMax=[]  IOutMin=[]  IOutMax=[]  DOutMin=[]  DOutMax=[]  NOutMin=[]  NOutMax=[]  SumOutMin=[]  SumOutMax=[]  SaturationOutMin=[]  SaturationOutMax=[]  PParamMin=[]  PParamMax=[]  IParamMin=[]  IParamMax=[]  DParamMin=[]  DParamMax=[]  NParamMin=[]  NParamMax=[]  KbParamMin=[]  KbParamMax=[]  KtParamMin=[]  KtParamMax=[]  KbOutMin=[]  KbOutMax=[]  KtOutMin=[]  KtOutMax=[]  IntegratorOutMin=[]  IntegratorOutMax=[]  FilterOutMin=[]  FilterOutMax=[]  SumI1OutMin=[]  SumI1OutMax=[]  SumI2OutMin=[]  SumI2OutMax=[]  SumI3OutMin=[]  SumI3OutMax=[]  SumI4OutMin=[]  SumI4OutMax=[]  SumDOutMin=[]  SumDOutMax=[]  DifferentiatorOutMin=[]  DifferentiatorOutMax=[]  FilterDiffOutCoefMin=[]  FilterDiffOutCoefMax=[]  ReciprocalOutMin=[]  ReciprocalOutMax=[]  SumDenOutMin=[]  SumDenOutMax=[]  SumNumOutMin=[]  SumNumOutMax=[]  DivideOutMin=[]  DivideOutMax=[]  UdiffTsProdOutMin=[]  UdiffTsProdOutMax=[]  NTsProdOutMin=[]  NTsProdOutMax=[]  UintegralTsProdOutMin=[]  UintegralTsProdOutMax=[]  UngainTsProdOutMin=[]  UngainTsProdOutMax=[]  IntegratorContinuousStateAttributes=''  IntegratorStateMustResolveToSignalObject=off  IntegratorRTWStateStorageClass=Auto  FilterContinuousStateAttributes=''  FilterStateMustResolveToSignalObject=off  FilterRTWStateStorageClass=Auto  ParallelPVariant=InternalParameters  IdealPVariant=Disabled  IVariant=InternalParameters  DVariant=InternalParameters  IntegratorVariant=Discrete  SatVariant=Disabled  AWVariant=Passthrough  PCopyVariant=Disabled  TRVariant=Disabled  FdbkBlocksVariant=Forward  IdealPFdbkVariant=Disabled  SatFdbkVariant=Disabled  DerivativeFilterVariant=ForwardEulerFilter  NVariant=InternalParameters  NCopyVariant=Disabled  FilterICVariant=InternalICsFilter  IntegratorICVariant=InternalICs  ExternalResetVariant=Disabled  TRSumVariant=Passthrough  SumFdbkVariant=Disabled  SumVariant=Sum_PID  TsampFilterVariant=InternalTs  TsampNgainVariant=Passthrough  TsampIntegralVariant=Passthrough  ExternalSaturationOutDataTypeStr=Inherit: Same as second input
  cfblk4 : simulink/Math Operations/Slider Gain  gain=1  low=0  high=2
  cfblk2 : Outport
  wires:
  cfblk4/1 -> cfblk3/1
  cfblk5/1 -> cfblk4/1
  cfblk7/1 -> cfblk2/1

== system sampleModel20/cfblk93 ==
  cfblk1 : Inport
  cfblk8 : Inport  Port=2
  cfblk3 : Sqrt  SaturateOnIntegerOverflow=on
  cfblk4 : ComplexToMagnitudeAngle
  cfblk5 : ComplexToRealImag
  cfblk6 : Subsystem
  cfblk7 : Subsystem
  cfblk9 : Delay  SampleTime=1
  cfblk2 : Outport
  wires:
  cfblk5/1 -> cfblk2/1
  cfblk7/1(cfblk2) -> cfblk3/1
  cfblk5/2 -> cfblk6/1(cfblk1)
  cfblk1/1 -> cfblk7/1(cfblk1)
  cfblk3/1 -> cfblk4/1
  cfblk8/1 -> cfblk7/2(cfblk11)
  cfblk4/1 -> cfblk5/1
  cfblk4/2 -> cfblk6/2(cfblk10)
  cfblk7/2(cfblk13) -> cfblk6/3(cfblk11)
  cfblk7/3(cfblk14) -> cfblk6/4(cfblk12)
  cfblk6/1(cfblk2) -> cfblk9/1
  cfblk9/1 -> cfblk7/3(cfblk12)

== system sampleModel20/cfblk94 ==
  cfblk1 : Inport
  cfblk12 : Inport  Port=2
  cfblk10 : Subsystem
  cfblk11 : Subsystem
  cfblk{14..19} (6 alike) : Delay  SampleTime=1
  cfblk3 : Product  Inputs=**
  cfblk4 : simulink/Math Operations/Slider Gain  gain=1  low=0  high=2
  cfblk5 : simulink/Math Operations/MinMax Running Resettable  Function=min  vinit=0.0
  cfblk6 : Subsystem
  cfblk7 : Subsystem
  cfblk8 : Subsystem
  cfblk9 : Subsystem
  cfblk2 : Outport
  cfblk13 : Outport  Port=2
  wires:
  cfblk8/1(cfblk2) -> cfblk9/1(cfblk1)
  cfblk1/1 -> cfblk10/1(cfblk1), cfblk6/2(cfblk9)
  cfblk5/1 -> cfblk13/1, cfblk7/1(cfblk1), cfblk7/3(cfblk6), cfblk7/5(cfblk8)
  cfblk10/1(cfblk2) -> cfblk3/1, cfblk7/2(cfblk5), cfblk7/4(cfblk7), cfblk3/2
  cfblk6/1(cfblk2) -> cfblk8/1(cfblk1)
  cfblk7/1(cfblk2) -> cfblk6/1(cfblk1), cfblk6/3(cfblk10)
  cfblk9/1(cfblk2) -> cfblk4/1
  cfblk6/2(cfblk11) -> cfblk8/5(cfblk13), cfblk19/1
  cfblk11/1(cfblk2) -> cfblk5/2, cfblk8/3(cfblk11)
  cfblk9/2(cfblk7) -> cfblk17/1, cfblk18/1
  cfblk4/1 -> cfblk14/1, cfblk15/1, cfblk16/1
  cfblk12/1 -> cfblk8/2(cfblk10)
  cfblk3/1 -> cfblk11/1(cfblk1), cfblk2/1, cfblk8/4(cfblk12)
  cfblk14/1 -> cfblk10/3(cfblk9)
  cfblk15/1 -> cfblk8/6(cfblk14)
  cfblk16/1 -> cfblk8/7(cfblk15)
  cfblk17/1 -> cfblk10/2(cfblk8)
  cfblk18/1 -> cfblk7/6(cfblk9)
  cfblk19/1 -> cfblk5/1

== system sampleModel20/cfblk95 ==
  cfblk1 : Inport
  cfblk12 : Inport  Port=2
  cfblk13 : Inport  Port=3
  cfblk10 : Subsystem
  cfblk11 : Subsystem
  cfblk{15..21} (7 alike) : Delay  SampleTime=1
  cfblk3 : Rounding
  cfblk4 : Sqrt  Operator=rSqrt  AlgorithmType=Newton-Raphson  SaturateOnIntegerOverflow=on
  cfblk5 : Trigonometry
  cfblk6 : Subsystem
  cfblk7 : Subsystem
  cfblk8 : Subsystem
  cfblk9 : Subsystem
  cfblk2 : Outport
  cfblk14 : Outport  Port=2
  wires:
  cfblk3/1 -> cfblk10/1(cfblk1)
  cfblk11/1(cfblk2) -> cfblk9/2(cfblk9), cfblk17/1
  cfblk4/1 -> cfblk14/1, cfblk8/1(cfblk1), cfblk11/1(cfblk1), cfblk7/6(cfblk10)
  cfblk9/1(cfblk2) -> cfblk2/1, cfblk18/1
  cfblk5/1 -> cfblk7/1(cfblk1)
  cfblk8/2(cfblk8) -> cfblk11/2(cfblk7), cfblk16/1
  cfblk10/1(cfblk2) -> cfblk6/1(cfblk1)
  cfblk1/1 -> cfblk3/1, cfblk7/3(cfblk7), cfblk7/4(cfblk8)
  cfblk12/1 -> cfblk7/2(cfblk6)
  cfblk10/2(cfblk14) -> cfblk5/1
  cfblk10/3(cfblk15) -> cfblk9/1(cfblk1)
  cfblk13/1 -> cfblk6/3(cfblk9), cfblk6/4(cfblk10)
  cfblk6/1(cfblk2) -> cfblk4/1, cfblk11/3(cfblk8), cfblk7/5(cfblk9)
  cfblk8/1(cfblk2) -> cfblk15/1
  cfblk15/1 -> cfblk10/2(cfblk8)
  cfblk16/1 -> cfblk10/5(cfblk11)
  cfblk17/1 -> cfblk10/3(cfblk9)
  cfblk18/1 -> cfblk10/4(cfblk10)
  cfblk7/1(cfblk2) -> cfblk19/1
  cfblk19/1 -> cfblk6/2(cfblk8)
  cfblk7/2(cfblk11) -> cfblk20/1
  cfblk20/1 -> cfblk10/6(cfblk12)
  cfblk7/3(cfblk12) -> cfblk21/1
  cfblk21/1 -> cfblk10/7(cfblk13)

== system sampleModel20/cfblk96 ==
  cfblk1 : Inport
  cfblk8 : Inport  Port=2
  cfblk9 : Inport  Port=3
  cfblk10 : Inport  Port=4
  cfblk11 : Delay  SampleTime=1
  cfblk12 : Delay  SampleTime=1
  cfblk3 : MinMax  Function=max
  cfblk4 : Constant  Value=[-604481834.839027]  SampleTime=1
  cfblk5 : Subsystem
  cfblk6 : Subsystem
  cfblk7 : Subsystem
  cfblk2 : Outport
  wires:
  cfblk4/1 -> cfblk7/1(cfblk1)
  cfblk3/1 -> cfblk5/5(cfblk12), cfblk5/6(cfblk13), cfblk11/1
  cfblk1/1 -> cfblk6/1(cfblk1)
  cfblk8/1 -> cfblk6/2(cfblk6), cfblk5/3(cfblk10), cfblk5/4(cfblk11)
  cfblk9/1 -> cfblk6/4(cfblk8)
  cfblk10/1 -> cfblk5/1(cfblk1)
  cfblk7/1(cfblk2) -> cfblk3/1
  cfblk6/1(cfblk2) -> cfblk2/1
  cfblk6/2(cfblk9) -> cfblk7/3(cfblk10), cfblk5/2(cfblk9)
  cfblk11/1 -> cfblk7/2(cfblk9)
  cfblk5/1(cfblk2) -> cfblk12/1
  cfblk12/1 -> cfblk6/3(cfblk7)

== system sampleModel20/cfblk97 ==
  cfblk1 : Inport
  cfblk5 : Inport  Port=2
  cfblk6 : Inport  Port=3
  cfblk3 : Subsystem
  cfblk4 : Subsystem
  cfblk8 : Delay  SampleTime=1
  cfblk2 : Outport
  cfblk7 : Outport  Port=2
  wires:
  cfblk4/1(cfblk2) -> cfblk2/1, cfblk3/4(cfblk13)
  cfblk3/1(cfblk2) -> cfblk7/1
  cfblk1/1 -> cfblk4/1(cfblk1)
  cfblk5/1 -> cfblk3/1(cfblk1), cfblk3/2(cfblk11), cfblk3/5(cfblk14)
  cfblk6/1 -> cfblk4/2(cfblk7), cfblk3/3(cfblk12)
  cfblk3/2(cfblk15) -> cfblk8/1
  cfblk8/1 -> cfblk4/3(cfblk8)

== system sampleModel20/cfblk98 ==
  cfblk1 : Inport
  cfblk10 : Inport  Port=2
  cfblk11 : Inport  Port=3
  cfblk3 : simulink/Discrete/Transfer Fcn First Order  PoleZ=0.95  ICPrevOutput=0.0  DoSatur=off
  cfblk4 : Math  Operator=mod  SaturateOnIntegerOverflow=on
  cfblk5 : ComplexToRealImag
  cfblk6 : PermuteDimensions
  cfblk7 : Trigonometry
  cfblk8 : Polyval  Coefs=[ +2.081618890e-019, -1.441693666e-014, +4.719686976e-010, -8.536869453e-006, +1.621573104e-001, -8.087801117e+001 ]
  cfblk9 : UnaryMinus
  cfblk2 : Outport
  cfblk12 : Outport  Port=2
  wires:
  cfblk1/1 -> cfblk4/1
  cfblk6/1 -> cfblk5/1
  cfblk3/1 -> cfblk2/1
  cfblk9/1 -> cfblk12/1
  cfblk5/1 -> cfblk9/1
  cfblk4/1 -> cfblk3/1
  cfblk11/1 -> cfblk8/1
  cfblk10/1 -> cfblk4/2
  cfblk8/1 -> cfblk7/1
  cfblk7/1 -> cfblk6/1

== system sampleModel20/cfblk99 ==
  cfblk1 : Inport
  cfblk8 : Inport  Port=2
  cfblk9 : Inport  Port=3
  cfblk10 : Inport  Port=4
  cfblk3 : simulink/Math Operations/Slider Gain  gain=1  low=0  high=2
  cfblk4 : UnaryMinus
  cfblk5 : simulink/Math Operations/MinMax Running Resettable  Function=min  vinit=0.0
  cfblk6 : Sin  TimeSource=Use external signal  SampleTime=0
  cfblk7 : Squeeze
  cfblk2 : Outport
  wires:
  cfblk7/1 -> cfblk2/1
  cfblk9/1 -> cfblk3/1
  cfblk6/1 -> cfblk5/1
  cfblk8/1 -> cfblk4/1
  cfblk3/1 -> cfblk6/1
  cfblk10/1 -> cfblk7/1
  cfblk1/1 -> cfblk5/2

== system sampleModel20/cfblk100/cfblk10 ==
  cfblk1 : Inport
  cfblk4 : Inport  Port=2
  cfblk5 : Inport  Port=3
  cfblk3 : Abs
  cfblk2 : Outport
  cfblk6 : Outport  Port=2
  cfblk7 : Outport  Port=3
  wires:
  cfblk4/1 -> cfblk2/1
  cfblk5/1 -> cfblk6/1
  cfblk1/1 -> cfblk3/1
  cfblk3/1 -> cfblk7/1

== system sampleModel20/cfblk100/cfblk11 ==
  cfblk1 : Inport
  cfblk9 : Inport  Port=2
  cfblk10 : Delay  SampleTime=1
  cfblk11 : Delay  SampleTime=1
  cfblk3 : Sum  Inputs=+
  cfblk4 : PermuteDimensions
  cfblk5 : Abs
  cfblk6 : Signum
  cfblk7 : Subsystem
  cfblk8 : Subsystem
  cfblk2 : Outport
  wires:
  cfblk6/1 -> cfblk3/1
  cfblk3/1 -> cfblk5/1
  cfblk4/1 -> cfblk8/1(cfblk1)
  cfblk9/1 -> cfblk2/1
  cfblk1/1 -> cfblk4/1, cfblk8/3(cfblk10)
  cfblk7/1(cfblk2) -> cfblk6/1
  cfblk5/1 -> cfblk10/1, cfblk11/1
  cfblk8/1(cfblk2) -> cfblk7/1(cfblk1)
  cfblk8/2(cfblk11) -> cfblk7/2(cfblk7)
  cfblk10/1 -> cfblk8/2(cfblk9)
  cfblk11/1 -> cfblk7/3(cfblk8)

== system sampleModel20/cfblk100/cfblk7 ==
  cfblk1 : Inport
  cfblk4 : Inport  Port=2
  cfblk5 : Inport  Port=3
  cfblk6 : Inport  Port=4
  cfblk7 : Inport  Port=5
  cfblk8 : Inport  Port=6
  cfblk3 : Signum
  cfblk2 : Outport
  wires:
  cfblk7/1 -> cfblk3/1
  cfblk8/1 -> cfblk2/1

== system sampleModel20/cfblk100/cfblk8 ==
  cfblk1 : Inport
  cfblk11 : Inport  Port=2
  cfblk12 : Inport  Port=3
  cfblk10 : Subsystem
  cfblk{13..20} (8 alike) : Delay  SampleTime=1
  cfblk3 : DiscreteIntegrator  ICPrevOutput=DiscIntNeverNeededParam  ICPrevScaledInput=DiscIntNeverNeededParam
  cfblk4 : Assignment  DiagnosticForDimensions=Warning  IndexOptions=Index vector (dialog)  Indices=1  OutputSizes=1
  cfblk5 : Signum
  cfblk6 : Subsystem
  cfblk7 : Subsystem
  cfblk8 : Subsystem
  cfblk9 : Subsystem
  cfblk2 : Outport
  wires:
  cfblk10/1(cfblk2) -> cfblk5/1
  cfblk1/1 -> cfblk9/1(cfblk1), cfblk8/5(cfblk12), cfblk10/2(cfblk11), cfblk10/5(cfblk14), cfblk9/5(cfblk12)
  cfblk9/1(cfblk2) -> cfblk3/1, cfblk4/2
  cfblk3/1 -> cfblk6/1(cfblk1), cfblk7/2(cfblk7), cfblk6/4(cfblk8), cfblk8/6(cfblk13), cfblk10/4(cfblk13), cfblk20/1
  cfblk4/1 -> cfblk10/6(cfblk15), cfblk17/1, cfblk18/1
  cfblk11/1 -> cfblk7/1(cfblk1)
  cfblk7/1(cfblk2) -> cfblk6/2(cfblk6)
  cfblk5/1 -> cfblk13/1, cfblk14/1, cfblk15/1, cfblk16/1
  cfblk8/1(cfblk2) -> cfblk10/1(cfblk1)
  cfblk8/2(cfblk14) -> cfblk4/1, cfblk2/1, cfblk19/1
  cfblk12/1 -> cfblk6/3(cfblk7), cfblk7/3(cfblk8), cfblk7/4(cfblk9)
  cfblk6/1(cfblk2) -> cfblk8/3(cfblk10), cfblk10/7(cfblk16)
  cfblk13/1 -> cfblk8/2(cfblk9)
  cfblk14/1 -> cfblk8/4(cfblk11)
  cfblk15/1 -> cfblk6/5(cfblk9)
  cfblk16/1 -> cfblk10/3(cfblk12)
  cfblk17/1 -> cfblk8/1(cfblk1)
  cfblk18/1 -> cfblk9/4(cfblk11)
  cfblk19/1 -> cfblk9/2(cfblk9)
  cfblk20/1 -> cfblk9/3(cfblk10)

== system sampleModel20/cfblk100/cfblk9 ==
  cfblk1 : Inport
  cfblk10 : Inport  Port=2
  cfblk11 : Inport  Port=3
  cfblk{13..17} (5 alike) : Delay  SampleTime=1
  cfblk3 : Product
  cfblk4 : Product  Inputs=**
  cfblk5 : DotProduct  InputSameDT=on  OutDataTypeStr=Inherit: Inherit via internal rule
  cfblk6 : Subsystem
  cfblk7 : Subsystem
  cfblk8 : Subsystem
  cfblk9 : Subsystem
  cfblk2 : Outport
  cfblk12 : Outport  Port=2
  wires:
  cfblk3/1 -> cfblk12/1, cfblk13/1
  cfblk11/1 -> cfblk2/1, cfblk3/2, cfblk6/2(cfblk14), cfblk8/6(cfblk12), cfblk6/3(cfblk15), cfblk7/6(cfblk14)
  cfblk1/1 -> cfblk8/3(cfblk9), cfblk8/8(cfblk14)
  cfblk7/1(cfblk2) -> cfblk4/1
  cfblk9/1(cfblk2) -> cfblk4/2, cfblk7/2(cfblk10), cfblk6/1(cfblk1), cfblk6/4(cfblk16)
  cfblk8/1(cfblk2) -> cfblk3/1, cfblk7/3(cfblk11), cfblk9/2(cfblk11), cfblk7/4(cfblk12)
  cfblk5/1 -> cfblk7/1(cfblk1), cfblk9/1(cfblk1), cfblk9/3(cfblk12)
  cfblk10/1 -> cfblk5/1, cfblk5/2, cfblk8/7(cfblk13)
  cfblk6/1(cfblk2) -> cfblk7/5(cfblk13), cfblk16/1, cfblk17/1
  cfblk13/1 -> cfblk8/2(cfblk8)
  cfblk4/1 -> cfblk14/1
  cfblk14/1 -> cfblk8/1(cfblk1)
  cfblk7/2(cfblk15) -> cfblk15/1
  cfblk15/1 -> cfblk8/4(cfblk10)
  cfblk16/1 -> cfblk8/5(cfblk11)
  cfblk17/1 -> cfblk9/4(cfblk13)

== system sampleModel20/cfblk77/cfblk10 ==
  cfblk1 : Inport
  cfblk8 : Inport  Port=2
  cfblk10 : Delay  SampleTime=1
  cfblk3 : Rounding
  cfblk4 : MinMax  Function=max  Inputs=2
  cfblk5 : Product  Inputs=*
  cfblk6 : Subsystem
  cfblk7 : Subsystem
  cfblk9 : Delay  SampleTime=1
  cfblk2 : Outport
  wires:
  cfblk7/1(cfblk2) -> cfblk5/1, cfblk4/2, cfblk6/2(cfblk7)
  cfblk3/1 -> cfblk4/1
  cfblk1/1 -> cfblk7/2(cfblk13)
  cfblk5/1 -> cfblk6/1(cfblk1)
  cfblk8/1 -> cfblk3/1, cfblk7/4(cfblk15)
  cfblk4/1 -> cfblk2/1, cfblk10/1
  cfblk6/1(cfblk2) -> cfblk9/1
  cfblk9/1 -> cfblk7/1(cfblk1)
  cfblk10/1 -> cfblk7/3(cfblk14)

== system sampleModel20/cfblk77/cfblk4 ==
  cfblk1 : Inport
  cfblk7 : Inport  Port=2
  cfblk8 : Inport  Port=3
  cfblk{9..12} (4 alike) : Delay  SampleTime=1
  cfblk3 : Product  Inputs=*
  cfblk4 : Sqrt  SaturateOnIntegerOverflow=on
  cfblk5 : Subsystem
  cfblk6 : Subsystem
  cfblk2 : Outport
  wires:
  cfblk8/1 -> cfblk2/1
  cfblk7/1 -> cfblk3/1
  cfblk1/1 -> cfblk6/1(cfblk1)
  cfblk4/1 -> cfblk9/1, cfblk10/1
  cfblk5/1(cfblk2) -> cfblk4/1
  cfblk3/1 -> cfblk6/2(cfblk10), cfblk5/5(cfblk10)
  cfblk6/1(cfblk2) -> cfblk5/2(cfblk7)
  cfblk6/2(cfblk14) -> cfblk5/3(cfblk8)
  cfblk6/3(cfblk15) -> cfblk5/4(cfblk9)
  cfblk9/1 -> cfblk5/1(cfblk1)
  cfblk10/1 -> cfblk6/5(cfblk13)
  cfblk5/2(cfblk11) -> cfblk11/1
  cfblk11/1 -> cfblk6/3(cfblk11)
  cfblk5/3(cfblk12) -> cfblk12/1
  cfblk12/1 -> cfblk6/4(cfblk12)

== system sampleModel20/cfblk77/cfblk5 ==
  cfblk1 : Inport
  cfblk11 : Inport  Port=2
  cfblk12 : Inport  Port=3
  cfblk13 : Inport  Port=4
  cfblk14 : Inport  Port=5
  cfblk15 : Inport  Port=6
  cfblk10 : Subsystem
  cfblk18 : Delay  SampleTime=1
  cfblk19 : Delay  SampleTime=1
  cfblk3 : Polyval  Coefs=[ +2.081618890e-019, -1.441693666e-014, +4.719686976e-010, -8.536869453e-006, +1.621573104e-001, -8.087801117e+001 ]
  cfblk4 : Gain  Gain=[-924803343.225796]
  cfblk5 : Abs
  cfblk6 : Product
  cfblk7 : MinMax  Function=max  Inputs=3
  cfblk8 : Subsystem
  cfblk9 : Subsystem
  cfblk2 : Outport
  cfblk16 : Outport  Port=2
  cfblk17 : Outport  Port=3
  wires:
  cfblk4/1 -> cfblk16/1, cfblk8/2(cfblk12)
  cfblk3/1 -> cfblk9/1(cfblk1)
  cfblk12/1 -> cfblk5/1
  cfblk14/1 -> cfblk3/1
  cfblk6/1 -> cfblk17/1, cfblk8/3(cfblk13)
  cfblk13/1 -> cfblk9/3(cfblk14)
  cfblk15/1 -> cfblk8/1(cfblk1)
  cfblk9/1(cfblk2) -> cfblk10/1(cfblk1)
  cfblk9/2(cfblk16) -> cfblk7/1
  cfblk11/1 -> cfblk7/2, cfblk6/2, cfblk10/3(cfblk15)
  cfblk1/1 -> cfblk2/1
  cfblk10/1(cfblk2) -> cfblk7/3
  cfblk10/2(cfblk16) -> cfblk4/1
  cfblk5/1 -> cfblk6/1, cfblk10/2(cfblk14)
  cfblk7/1 -> cfblk18/1
  cfblk18/1 -> cfblk9/4(cfblk15)
  cfblk8/1(cfblk2) -> cfblk19/1
  cfblk19/1 -> cfblk9/2(cfblk13)

== system sampleModel20/cfblk77/cfblk6 ==
  cfblk1 : Inport
  cfblk10 : Inport  Port=2
  cfblk11 : Inport  Port=3
  cfblk12 : Inport  Port=4
  cfblk13 : Inport  Port=5
  cfblk{14..21} (8 alike) : Delay  SampleTime=1
  cfblk3 : Polyval  Coefs=[ +2.081618890e-019, -1.441693666e-014, +4.719686976e-010, -8.536869453e-006, +1.621573104e-001, -8.087801117e+001 ]
  cfblk4 : Assignment  DiagnosticForDimensions=Warning  IndexOptions=Index vector (dialog)  Indices=1  OutputSizes=1
  cfblk5 : Subsystem
  cfblk6 : Subsystem
  cfblk7 : Subsystem
  cfblk8 : Subsystem
  cfblk9 : Subsystem
  cfblk2 : Outport
  wires:
  cfblk13/1 -> cfblk4/1, cfblk8/4(cfblk12), cfblk8/7(cfblk15), cfblk8/9(cfblk17)
  cfblk7/1(cfblk2) -> cfblk8/1(cfblk1), cfblk8/3(cfblk11), cfblk6/6(cfblk13), cfblk8/8(cfblk16)
  cfblk8/1(cfblk2) -> cfblk6/1(cfblk1), cfblk21/1
  cfblk12/1 -> cfblk7/1(cfblk1), cfblk8/6(cfblk14)
  cfblk5/2(cfblk13) -> cfblk9/1(cfblk1)
  cfblk4/1 -> cfblk6/2(cfblk9)
  cfblk5/3(cfblk14) -> cfblk2/1
  cfblk5/4(cfblk15) -> cfblk9/2(cfblk9)
  cfblk11/1 -> cfblk6/3(cfblk10)
  cfblk1/1 -> cfblk7/2(cfblk13)
  cfblk10/1 -> cfblk4/2
  cfblk9/2(cfblk10) -> cfblk3/1, cfblk18/1
  cfblk6/2(cfblk14) -> cfblk5/2(cfblk10)
  cfblk6/3(cfblk15) -> cfblk5/3(cfblk11)
  cfblk6/5(cfblk17) -> cfblk5/4(cfblk12), cfblk20/1
  cfblk6/1(cfblk2) -> cfblk14/1
  cfblk14/1 -> cfblk7/3(cfblk14)
  cfblk5/1(cfblk2) -> cfblk15/1
  cfblk15/1 -> cfblk8/2(cfblk10)
  cfblk9/1(cfblk2) -> cfblk16/1
  cfblk16/1 -> cfblk6/4(cfblk11)
  cfblk3/1 -> cfblk17/1
  cfblk17/1 -> cfblk5/1(cfblk1)
  cfblk18/1 -> cfblk6/5(cfblk12)
  cfblk6/4(cfblk16) -> cfblk19/1
  cfblk19/1 -> cfblk7/4(cfblk15)
  cfblk20/1 -> cfblk8/5(cfblk13)
  cfblk21/1 -> cfblk7/5(cfblk16)

== system sampleModel20/cfblk77/cfblk7 ==
  cfblk1 : Inport
  cfblk11 : Inport  Port=2
  cfblk10 : Subsystem
  cfblk{12..17} (6 alike) : Delay  SampleTime=1
  cfblk3 : Sum  Inputs=-+
  cfblk4 : simulink/Math Operations/Slider Gain  gain=1  low=0  high=2
  cfblk5 : Abs
  cfblk6 : PermuteDimensions
  cfblk7 : Assignment  DiagnosticForDimensions=Warning  IndexOptions=Index vector (dialog)  Indices=1  OutputSizes=1
  cfblk8 : Subsystem
  cfblk9 : Subsystem
  cfblk2 : Outport
  wires:
  cfblk1/1 -> cfblk3/1, cfblk10/3(cfblk15)
  cfblk9/1(cfblk2) -> cfblk5/1
  cfblk3/1 -> cfblk8/1(cfblk1), cfblk9/5(cfblk14)
  cfblk11/1 -> cfblk2/1, cfblk9/3(cfblk12)
  cfblk9/3(cfblk17) -> cfblk4/1
  cfblk7/1 -> cfblk6/1, cfblk9/4(cfblk13), cfblk13/1
  cfblk10/1(cfblk2) -> cfblk7/2
  cfblk8/1(cfblk2) -> cfblk10/2(cfblk14), cfblk9/6(cfblk15)
  cfblk10/2(cfblk16) -> cfblk9/2(cfblk11), cfblk17/1
  cfblk6/1 -> cfblk12/1
  cfblk12/1 -> cfblk8/2(cfblk10)
  cfblk13/1 -> cfblk3/2
  cfblk5/1 -> cfblk14/1
  cfblk14/1 -> cfblk9/1(cfblk1)
  cfblk9/2(cfblk16) -> cfblk15/1
  cfblk15/1 -> cfblk7/1
  cfblk4/1 -> cfblk16/1
  cfblk16/1 -> cfblk10/1(cfblk1)
  cfblk17/1 -> cfblk8/3(cfblk11)

== system sampleModel20/cfblk77/cfblk8 ==
  cfblk1 : Inport
  cfblk11 : Inport  Port=2
  cfblk12 : Inport  Port=3
  cfblk13 : Inport  Port=4
  cfblk10 : Subsystem
  cfblk{16..19} (4 alike) : Delay  SampleTime=1
  cfblk3 : Sum  Inputs=+
  cfblk4 : Squeeze
  cfblk5 : Subsystem
  cfblk6 : Subsystem
  cfblk7 : Subsystem
  cfblk8 : Subsystem
  cfblk9 : Subsystem
  cfblk2 : Outport
  cfblk14 : Outport  Port=2
  cfblk15 : Outport  Port=3
  wires:
  cfblk9/1(cfblk2) -> cfblk3/1
  cfblk4/1 -> cfblk7/1(cfblk1)
  cfblk9/2(cfblk10) -> cfblk15/1
  cfblk5/1(cfblk2) -> cfblk14/1
  cfblk7/1(cfblk2) -> cfblk5/1(cfblk1)
  cfblk10/1(cfblk2) -> cfblk6/1(cfblk1)
  cfblk12/1 -> cfblk10/1(cfblk1)
  cfblk7/2(cfblk11) -> cfblk10/2(cfblk9), cfblk9/2(cfblk7), cfblk10/4(cfblk11), cfblk9/4(cfblk9)
  cfblk1/1 -> cfblk8/1(cfblk1), cfblk5/2(cfblk9)
  cfblk13/1 -> cfblk8/2(cfblk11), cfblk10/5(cfblk12)
  cfblk6/1(cfblk2) -> cfblk2/1, cfblk5/3(cfblk10), cfblk16/1
  cfblk11/1 -> cfblk8/4(cfblk13), cfblk6/2(cfblk11)
  cfblk8/1(cfblk2) -> cfblk4/1
  cfblk3/1 -> cfblk18/1, cfblk19/1
  cfblk16/1 -> cfblk10/3(cfblk10)
  cfblk10/2(cfblk13) -> cfblk17/1
  cfblk17/1 -> cfblk8/3(cfblk12)
  cfblk18/1 -> cfblk9/1(cfblk1)
  cfblk19/1 -> cfblk9/3(cfblk8)
